simulink model "sliderCrank"  (R2023a)
settings: Solver=VariableStepAuto  StartTime=0.0  StopTime=10.0  RelTol=1e-3
libraries: simulink x1
settings Model: Creator=saidb  LastModifiedBy=saidb

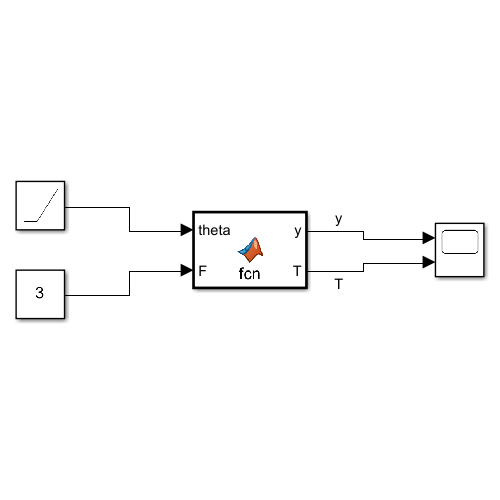
[thumbnail: Simulink's stored preview of the top-level diagram]
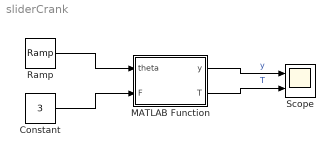
== system sliderCrank ==
  Constant : Constant  Value=3
  MATLAB Function : MATLAB Function  TreatAsAtomicUnit=on
  Ramp : simulink/Sources/Ramp  slope=1  start=0  InitialOutput=0
  Scope : Scope  NumInputPorts=2
  wires:
  Ramp/1 -> MATLAB Function/1(theta)
  MATLAB Function/1(y) -> Scope/1  "y"
  MATLAB Function/2(T) -> Scope/2  "T"
  Constant/1 -> MATLAB Function/2(F)

== matlab function sliderCrank/MATLAB Function ==
  data: theta input; y output; F input; T output
function [y,T] = fcn(theta, F)

l1 = 0.05;
l2 = 0.1;
e = 0;
h = 0;
gamma = abs(asin((l1 * sin(theta) + e) / (l2)));
beta = pi - theta - gamma;

y = sqrt(l2^2 - (l1 * sin(theta) + e)^2) + l1 * cos(theta) + h;
T = F * cos(gamma) * sin(pi - beta) * l1;
